simulink library "PC_Simulator_Lib"  (Simulink 8.2)
settings: Solver=ode45  StartTime=0.0  StopTime=10.0  RelTol=1e-3
values from neighbouring files (symbols this model uses):
  data = [r1 r2 r3 r4 L1 L2 L3 L4]    [strasse_Bedatung_HNI_ITI.m]
  distSameLane = 60    [InitialisationsEnv.m]
  eng_speed = [0 60 120 180 240 300 360 420 480 540 600 660 ... (101 elements, 1x101)]    [engine_table.mat]    (also in motor_parameter_calc.m = omega)
  Heading_init = 0    [Start.m]
  inertiaLateral = 25*(radiusWheel)^2    (= 4.129024)    [Start.m]
  laneWidth = 3.6    [InitialisationsEnv.m]    (also in strasse_Bedatung_HNI_ITI.m)
  omega_engine = [0.000000 150.000000 500.000000 1000.000000 1500.000000 2000.000000 2500.000000 3000.000000 3500.000000 4000.000000 4500.000000 5000.000000 5500.000000 6000.000000]    [friction_tables.m]
  omega_max = 6000    [engine_table.mat]    (also in motor_parameter_calc.m)
  omega_wheel = [0 20 40 60 80 100 122 143.7 164]    [friction_tables.m]
  para_Fellow_8_Points = ADAS.Fellow_8_Points    [ADAS_parameters.m]
  position_start_x = [x1 x2 x3 x4 x5 x6 x7]    [strasse_Bedatung_HNI_ITI.m]
  position_start_y = [y1 y2 y3 y4 y5 y6 y7]    [strasse_Bedatung_HNI_ITI.m]
  rad3rdLine = 57.2    [InitialisationsEnv.m]    (also in strasse_Bedatung_HNI_ITI.m)
  radiusWheel = 16*2.54/100    (= 0.4064)    [Start.m]
  s_values = [S1 S2 S3 S4 S5 S6 S7]    [strasse_Bedatung_HNI_ITI.m]
  segmentLimits = [segment1EndThirdLine                   segment2EndThirdLine                   segment3EndThirdLine                   segment4EndThirdLine                   segment5EndThirdLine                   segment6EndThirdLine                   segment7EndThirdLine                   segment8EndThirdLine                   ]    [InitialisationsEnv.m]    (also in strasse_Bedatung_HNI_ITI.m)
  setPosT = [-1.8 -5.4 -1.8 -5.4 -1.8 -5.4 -1.8 -5.4 -1.8 -5.4]    [InitialisationsEnv.m]
  torque = [297.089227105 300.997600937 304.800343044 308.497453426 312.088932082 315.574779014 318.95499422 322.229577701 325.398529457 328.461849487 331.419537793 334.271594373 ... (101 elements, 1x101)]    [engine_table.mat]    (also in motor_parameter_calc.m = g)
  Torque_lost = [0.000000 -8.777780 -15.000000 -26.800000 -29.600000 -32.700000 -35.900000 -39.300000 -42.800000 -46.500000 -50.300000 -54.300000 -58.500000 -62.800000 ]*0.6    [friction_tables.m]
  Torque_lost_wheel = [0.8 0.8 0.75 0.7 0.4 0.3 0.2 0.07 0.07]*0.2    [friction_tables.m]
  X_init = 0    [Start.m]
  Y_init = 1.8    [Start.m]
  Z_init = 0    [Start.m]
undefined symbols (not defined in the file or in its folder): Acc_Pedal, ADAS, Brake_Pedal, Joystick, Newton, Para, Raphson, Standard_Devices, Steering_Wheel_Angle, UDP_Protocol
libraries: simulink x43, rtwinlib x7, dspnetwork x2, simulink_extras x1, vrlib x1
(part 7 of 13)

== system PC_Simulator_Lib/Comunication_with_visualisation_normal_mode_new_Version/Subsystem2/Subsystem7 ==
  In1 : Inport
  Constant9 : Constant  Value=Z_init
  Sum : Sum  Inputs=|++
  Out1 : Outport
  wires:
  Sum/1 -> Out1/1
  Constant9/1 -> Sum/2
  In1/1 -> Sum/1

== system PC_Simulator_Lib/Comunication_with_visualisation_normal_mode_new_Version/Subsystem2/Subsystem8 ==
  In1 : Inport
  Constant9 : Constant  Value=Z_init
  Sum : Sum  Inputs=|++
  Out1 : Outport
  wires:
  In1/1 -> Sum/1
  Constant9/1 -> Sum/2
  Sum/1 -> Out1/1

== system PC_Simulator_Lib/Comunication_with_visualisation_normal_mode_new_Version/Subsystem2/Subsystem9 ==
  In1 : Inport
  Constant9 : Constant  Value=Z_init
  Sum : Sum  Inputs=|++
  Out1 : Outport
  wires:
  Sum/1 -> Out1/1
  Constant9/1 -> Sum/2
  In1/1 -> Sum/1

== system PC_Simulator_Lib/Drive_Train/4_Wheels_drive_train_and_Brake/Brake ==
  Feedback : Inport
  Add : Sum
  Bus Selector1 : BusSelector  OutputSignals=Vehicle_Dynamics.Vx_COG[m|s]
  Bus Selector6 : BusSelector  OutputSignals=ADAS.Brake_Pedal[norm]
  Compare To Constant : simulink/Logic and Bit Operations/Compare To Constant  relop=>=  const=0.7  OutDataTypeStr=uint8
  Compare To Constant1 : simulink/Logic and Bit Operations/Compare To Constant  relop=<=  const=-1  OutDataTypeStr=uint8
  Compare To Constant2 : simulink/Logic and Bit Operations/Compare To Constant  relop=<  const=0  OutDataTypeStr=uint8
  Constant1 : Constant  Value=0.35
  Constant2 : Constant
  Data Type Conversion : DataTypeConversion
  Data Type Conversion1 : DataTypeConversion
  Ground : Ground
  Ground1 : Ground
  Logical Operator : Logic  Operator=OR  AllPortsSameDT=off  OutDataTypeStr=boolean
  Product : Product  Inputs=5  RndMeth=Zero
  Product1 : Product  RndMeth=Zero
  Saturation : Saturate  UpperLimit=1  LowerLimit=0
  Sign : Signum
  Subsystem : Subsystem
  Subsystem1 : Subsystem
  Switch : Switch  Criteria=u2 > Threshold
  Terminator : Terminator
  Torque_max : Constant  Value=Para.DT.Torque_max_Brake.v
  Torque_Brake_Nm : Outport
  wires:
  Ground1/1 -> Subsystem/2(Omega_rad/s)
  Ground/1 -> Subsystem/1(Torque_Brake_Nm)
  Subsystem/1(Torque_Brake_act_Nm) -> Terminator/1
  Logical Operator/1 -> Data Type Conversion/1
  Compare To Constant/1 -> Logical Operator/1
  Bus Selector6/1 -> Saturation/1  "<Brake_Pedal[norm]>"
  Sign/1 -> Product/2
  Bus Selector1/1 -> Compare To Constant/1, Compare To Constant1/1, Subsystem1/1(v_X_CoG[m|s]), Compare To Constant2/1, Sign/1  "<Vx_COG[m|s]>"
  Feedback/1 -> Bus Selector1/1, Bus Selector6/1
  Torque_max/1 -> Product1/1
  Saturation/1 -> Product1/2, Subsystem1/2(Brake_Pedal[norm])
  Compare To Constant2/1 -> Data Type Conversion1/1
  Data Type Conversion1/1 -> Switch/2
  Constant1/1 -> Switch/1
  Product1/1 -> Product/1
  Switch/1 -> Product/4
  Constant2/1 -> Product/5, Switch/3
  Data Type Conversion/1 -> Product/3
  Compare To Constant1/1 -> Logical Operator/2
  Product/1 -> Add/1
  Add/1 -> Torque_Brake_Nm/1
  Subsystem1/1(Out1) -> Add/2

== system PC_Simulator_Lib/Drive_Train/4_Wheels_drive_train_and_Brake/FL ==
  F_z : Inport
  Vx : Inport  Port=2
  Vy : Inport  Port=3
  Coeffecient_of_friction : Inport  Port=4
  Torque_Drive_Nm : Inport  Port=5
  Torque_Brake_Nm : Inport  Port=6
  Alpha_Kappa_Selector2 : Subsystem
  Fx_calculator : MATLAB Function  TreatAsAtomicUnit=on
  Fy_calculator : MATLAB Function  TreatAsAtomicUnit=on
  Radius_of_tire : Constant  Value=radiusWheel
  Wheel dynamics : Subsystem
  Fx : Outport
  Fy : Outport  Port=2
  Omega : Outport  Port=3
  omegaDot_radPs2 : Outport  Port=4
  wires:
  Wheel dynamics/1(omega_radPs) -> Omega/1, Alpha_Kappa_Selector2/3(omega)
  Vx/1 -> Fy_calculator/3(V_x), Alpha_Kappa_Selector2/1(Vx)
  Radius_of_tire/1 -> Alpha_Kappa_Selector2/4(Rdyn)
  Vy/1 -> Alpha_Kappa_Selector2/2(Vy)
  F_z/1 -> Fy_calculator/4(Fz), Fx_calculator/3(Fz)
  Fy_calculator/1(Fy) -> Fy/1
  Coeffecient_of_friction/1 -> Fy_calculator/5(mue), Fx_calculator/4(mue)
  Fx_calculator/1(Fx) -> Wheel dynamics/1(F_x), Fx/1, Alpha_Kappa_Selector2/5(Fx)  "F_long"
  Wheel dynamics/2(omegaDot_radPs2) -> omegaDot_radPs2/1
  Torque_Drive_Nm/1 -> Wheel dynamics/2(Torque_Drive_Nm)
  Torque_Brake_Nm/1 -> Wheel dynamics/3(Torque_Brake_Nm)
  Alpha_Kappa_Selector2/1(kappa) -> Fx_calculator/1(lambda), Fy_calculator/1(lambda)
  Alpha_Kappa_Selector2/2(alpha) -> Fy_calculator/2(alpha), Fx_calculator/2(alpha)

== system PC_Simulator_Lib/Drive_Train/4_Wheels_drive_train_and_Brake/FR ==
  F_z : Inport
  Vx : Inport  Port=2
  Vy : Inport  Port=3
  Coeffecient_of_friction : Inport  Port=4
  Torque_Drive_Nm : Inport  Port=5
  Torque_Brake_Nm : Inport  Port=6
  Alpha_Kappa_Selector2 : Subsystem
  Fx_calculator : MATLAB Function  TreatAsAtomicUnit=on
  Fy_calculator : MATLAB Function  TreatAsAtomicUnit=on
  Radius_of_tire : Constant  Value=radiusWheel
  Wheel dynamics : Subsystem
  Fx : Outport
  Fy : Outport  Port=2
  Omega : Outport  Port=3
  omegaDot_radPs2 : Outport  Port=4
  wires:
  Wheel dynamics/1(omega_radPs) -> Alpha_Kappa_Selector2/3(omega), Omega/1
  Vx/1 -> Alpha_Kappa_Selector2/1(Vx), Fy_calculator/3(V_x)
  Radius_of_tire/1 -> Alpha_Kappa_Selector2/4(Rdyn)
  Vy/1 -> Alpha_Kappa_Selector2/2(Vy)
  F_z/1 -> Fy_calculator/4(Fz), Fx_calculator/3(Fz)
  Alpha_Kappa_Selector2/2(alpha) -> Fx_calculator/2(alpha), Fy_calculator/2(alpha)
  Alpha_Kappa_Selector2/1(kappa) -> Fy_calculator/1(lambda), Fx_calculator/1(lambda)
  Fy_calculator/1(Fy) -> Fy/1
  Coeffecient_of_friction/1 -> Fy_calculator/5(mue), Fx_calculator/4(mue)
  Fx_calculator/1(Fx) -> Alpha_Kappa_Selector2/5(Fx), Wheel dynamics/1(F_x), Fx/1  "F_long"
  Wheel dynamics/2(omegaDot_radPs2) -> omegaDot_radPs2/1
  Torque_Drive_Nm/1 -> Wheel dynamics/2(Torque_Drive_Nm)
  Torque_Brake_Nm/1 -> Wheel dynamics/3(Torque_Brake_Nm)

== system PC_Simulator_Lib/Drive_Train/4_Wheels_drive_train_and_Brake/RL ==
  F_z : Inport
  Vx : Inport  Port=2
  Vy : Inport  Port=3
  Coeffecient_of_friction : Inport  Port=4
  Torque_Drive_Nm : Inport  Port=5
  Torque_Brake_Nm : Inport  Port=6
  Alpha_Kappa_Selector2 : Subsystem
  Fx_calculator : MATLAB Function  TreatAsAtomicUnit=on
  Fy_calculator : MATLAB Function  TreatAsAtomicUnit=on
  Radius_of_tire : Constant  Value=radiusWheel
  Wheel dynamics : Subsystem
  Fx : Outport
  Fy : Outport  Port=2
  Omega : Outport  Port=3
  omegaDot_radPs2 : Outport  Port=4
  wires:
  Wheel dynamics/1(omega_radPs) -> Omega/1, Alpha_Kappa_Selector2/3(omega)
  Vx/1 -> Alpha_Kappa_Selector2/1(Vx), Fy_calculator/3(V_x)
  Radius_of_tire/1 -> Alpha_Kappa_Selector2/4(Rdyn)
  Vy/1 -> Alpha_Kappa_Selector2/2(Vy)
  F_z/1 -> Fy_calculator/4(Fz), Fx_calculator/3(Fz)
  Alpha_Kappa_Selector2/2(alpha) -> Fx_calculator/2(alpha), Fy_calculator/2(alpha)
  Alpha_Kappa_Selector2/1(kappa) -> Fy_calculator/1(lambda), Fx_calculator/1(lambda)
  Fy_calculator/1(Fy) -> Fy/1
  Coeffecient_of_friction/1 -> Fy_calculator/5(mue), Fx_calculator/4(mue)
  Fx_calculator/1(Fx) -> Wheel dynamics/1(F_x), Fx/1, Alpha_Kappa_Selector2/5(Fx)  "F_long"
  Wheel dynamics/2(omegaDot_radPs2) -> omegaDot_radPs2/1
  Torque_Drive_Nm/1 -> Wheel dynamics/2(Torque_Drive_Nm)
  Torque_Brake_Nm/1 -> Wheel dynamics/3(Torque_Brake_Nm)

== system PC_Simulator_Lib/Drive_Train/4_Wheels_drive_train_and_Brake/RR ==
  F_z : Inport
  Vx : Inport  Port=2
  Vy : Inport  Port=3
  Coeffecient_of_friction : Inport  Port=4
  Torque_Drive_Nm : Inport  Port=5
  Torque_Brake_Nm : Inport  Port=6
  Alpha_Kappa_Selector2 : Subsystem
  Fx_calculator : MATLAB Function  TreatAsAtomicUnit=on
  Fy_calculator : MATLAB Function  TreatAsAtomicUnit=on
  Radius_of_tire : Constant  Value=radiusWheel
  Wheel dynamics : Subsystem
  Fx : Outport
  Fy : Outport  Port=2
  Omega : Outport  Port=3
  omegaDot_radPs2 : Outport  Port=4
  wires:
  Wheel dynamics/1(omega_radPs) -> Omega/1, Alpha_Kappa_Selector2/3(omega)
  Vx/1 -> Fy_calculator/3(V_x), Alpha_Kappa_Selector2/1(Vx)
  Radius_of_tire/1 -> Alpha_Kappa_Selector2/4(Rdyn)
  Vy/1 -> Alpha_Kappa_Selector2/2(Vy)
  F_z/1 -> Fy_calculator/4(Fz), Fx_calculator/3(Fz)
  Alpha_Kappa_Selector2/2(alpha) -> Fx_calculator/2(alpha), Fy_calculator/2(alpha)
  Alpha_Kappa_Selector2/1(kappa) -> Fy_calculator/1(lambda), Fx_calculator/1(lambda)
  Fy_calculator/1(Fy) -> Fy/1
  Coeffecient_of_friction/1 -> Fy_calculator/5(mue), Fx_calculator/4(mue)
  Fx_calculator/1(Fx) -> Wheel dynamics/1(F_x), Fx/1, Alpha_Kappa_Selector2/5(Fx)  "F_long"
  Wheel dynamics/2(omegaDot_radPs2) -> omegaDot_radPs2/1
  Torque_Drive_Nm/1 -> Wheel dynamics/2(Torque_Drive_Nm)
  Torque_Brake_Nm/1 -> Wheel dynamics/3(Torque_Brake_Nm)

== system PC_Simulator_Lib/Environment/Environment_Model/Master driver ==
  setVelS[km/h] : Inport
  setPosT[m] : Inport  Port=2
  actualPosS[m] : Inport  Port=3
  actualPosT[m] : Inport  Port=4
  actualVelS[m/s] : Inport  Port=5
  distSameLanes[m] : Inport  Port=6
  mainCarPosS[m] : Inport  Port=7
  mainCarPosT[m] : Inport  Port=8
  mainCarVelS[m/s] : Inport  Port=9
  mainCarWidth[m] : Inport  Port=10
  masterDriver : MATLAB Function  TreatAsAtomicUnit=on
  desiredVelS[km/h] : Outport
  desiredPosT[m] : Outport  Port=2
  wires:
  masterDriver/2(desiredPosT) -> desiredPosT[m]/1
  masterDriver/1(desiredVelS) -> desiredVelS[km/h]/1
  mainCarPosS[m]/1 -> masterDriver/7(mainCarPosS)
  distSameLanes[m]/1 -> masterDriver/6(distSameLanes)
  actualVelS[m/s]/1 -> masterDriver/5(actualVelS)
  actualPosT[m]/1 -> masterDriver/4(actualPosT)
  actualPosS[m]/1 -> masterDriver/3(actualPosS)
  setPosT[m]/1 -> masterDriver/2(setPosT)
  setVelS[km/h]/1 -> masterDriver/1(setVelS)
  mainCarPosT[m]/1 -> masterDriver/8(mainCarPosT)
  mainCarVelS[m/s]/1 -> masterDriver/9(mainCarVelS)
  mainCarWidth[m]/1 -> masterDriver/10(mainCarWidth)

== system PC_Simulator_Lib/Environment/Environment_Model/Road model ==
  note: Simple road model to transform the (s,t) point of the
      | local coordinate system to (x,y) point of the global
      | coordinate system
  note: Road model to transform
      | the (s,t) point to (x,y) point
  s[m] : Inport
  t[m] : Inport  Port=2
  segmentLimits[m] : Inport  Port=3
  laneWidth[m] : Inport  Port=4
  rad3rdLine[m] : Inport  Port=5
  st_xy : MATLAB Function  TreatAsAtomicUnit=on
  x[m] : Outport
  y[m] : Outport  Port=2
  z[m] : Outport  Port=3
  headingAngle[deg] : Outport  Port=4
  wires:
  st_xy/4(headingAngle) -> headingAngle[deg]/1
  st_xy/3(z) -> z[m]/1
  st_xy/2(y) -> y[m]/1
  st_xy/1(x) -> x[m]/1
  rad3rdLine[m]/1 -> st_xy/5(rad3rdLine)
  laneWidth[m]/1 -> st_xy/4(laneWidth)
  segmentLimits[m]/1 -> st_xy/3(segmentLimits)
  t[m]/1 -> st_xy/2(t)
  s[m]/1 -> st_xy/1(s)

== system PC_Simulator_Lib/Environment/Environment_Model/Subsystem ==
  v_relative_Sensor[m|s] : Inport
  1-D Lookup Table1 : Lookup_n-D  NumberOfTableDimensions=1  BreakpointsForDimension1=ADAS.EBA.Braking_Distance_LookUpTable.velocity  BeginIndexSearchUsingPreviousIndexResult=on  Table=ADAS.EBA.Braking_Distance_LookUpTable.Distance  InternalRulePriority=Speed  RndMeth=Simplest  InputSameDT=on
  Abs : Abs
  Divide : Product  Inputs=/*
  Gain : Gain  Gain=3.6
  Math Function : Math  Operator=square  SaturateOnIntegerOverflow=on
  Braking_Distance[m] : Outport
  wires:
  v_relative_Sensor[m|s]/1 -> Abs/1, Math Function/1
  Math Function/1 -> Divide/2
  Divide/1 -> Braking_Distance[m]/1
  Gain/1 -> 1-D Lookup Table1/1
  1-D Lookup Table1/1 -> Divide/1
  Abs/1 -> Gain/1

== system PC_Simulator_Lib/Environment/Environment_Model/Traffic_Vehicle_Model1 ==
  ResetSig[] : Inport
  VelSDesired : Inport  Port=2
  Vehicle_Model_s : Subsystem
  VelS[m/s] : Outport
  PosS[m] : Outport  Port=2
  wires:
  Vehicle_Model_s/1(VelS[m/s]) -> VelS[m/s]/1
  Vehicle_Model_s/2(PosS[m]) -> PosS[m]/1
  ResetSig[]/1 -> Vehicle_Model_s/1(ResetSig[])
  VelSDesired/1 -> Vehicle_Model_s/2(VelSDesired[Km/h])

== system PC_Simulator_Lib/Environment/Environment_Model/Traffic_Vehicle_Model11 ==
  ResetSig[] : Inport
  VelSDesired[km/h] : Inport  Port=2
  PosTDesired[m] : Inport  Port=3
  Vehicle_Model_s : Subsystem
  Vehicle_Model_t : Subsystem
  VelS[m/s] : Outport
  PosS[m] : Outport  Port=2
  PosT[m] : Outport  Port=3
  wires:
  PosTDesired[m]/1 -> Vehicle_Model_t/2(PosTDesired[m])
  Vehicle_Model_t/1(PosT[m]) -> PosT[m]/1
  VelSDesired[km/h]/1 -> Vehicle_Model_s/2(VelSDesired[Km/h])
  ResetSig[]/1 -> Vehicle_Model_t/1(ResetSig[]), Vehicle_Model_s/1(ResetSig[])
  Vehicle_Model_s/2(PosS[m]) -> PosS[m]/1
  Vehicle_Model_s/1(VelS[m/s]) -> VelS[m/s]/1

== system PC_Simulator_Lib/Environment/Environment_Model/Traffic_Vehicle_Model2 ==
  ResetSig[] : Inport
  VelSDesired : Inport  Port=2
  Vehicle_Model_s : Subsystem
  VelS[m/s] : Outport
  PosS[m] : Outport  Port=2
  wires:
  Vehicle_Model_s/1(VelS[m/s]) -> VelS[m/s]/1
  Vehicle_Model_s/2(PosS[m]) -> PosS[m]/1
  ResetSig[]/1 -> Vehicle_Model_s/1(ResetSig[])
  VelSDesired/1 -> Vehicle_Model_s/2(VelSDesired[Km/h])

== system PC_Simulator_Lib/Environment/Environment_Model/Traffic_Vehicle_Model3 ==
  ResetSig[] : Inport
  VelSDesired : Inport  Port=2
  Vehicle_Model_s : Subsystem
  VelS[m/s] : Outport
  PosS[m] : Outport  Port=2
  wires:
  Vehicle_Model_s/1(VelS[m/s]) -> VelS[m/s]/1
  Vehicle_Model_s/2(PosS[m]) -> PosS[m]/1
  ResetSig[]/1 -> Vehicle_Model_s/1(ResetSig[])
  VelSDesired/1 -> Vehicle_Model_s/2(VelSDesired[Km/h])

== system PC_Simulator_Lib/Environment/Environment_Model/Traffic_Vehicle_Model4 ==
  ResetSig[] : Inport
  VelSDesired : Inport  Port=2
  Vehicle_Model_s : Subsystem
  VelS[m/s] : Outport
  PosS[m] : Outport  Port=2
  wires:
  Vehicle_Model_s/1(VelS[m/s]) -> VelS[m/s]/1
  Vehicle_Model_s/2(PosS[m]) -> PosS[m]/1
  ResetSig[]/1 -> Vehicle_Model_s/1(ResetSig[])
  VelSDesired/1 -> Vehicle_Model_s/2(VelSDesired[Km/h])

== system PC_Simulator_Lib/Environment/Environment_Model/Traffic_Vehicle_Model5 ==
  ResetSig[] : Inport
  VelSDesired : Inport  Port=2
  Vehicle_Model_s : Subsystem
  VelS[m/s] : Outport
  PosS[m] : Outport  Port=2
  wires:
  Vehicle_Model_s/1(VelS[m/s]) -> VelS[m/s]/1
  Vehicle_Model_s/2(PosS[m]) -> PosS[m]/1
  ResetSig[]/1 -> Vehicle_Model_s/1(ResetSig[])
  VelSDesired/1 -> Vehicle_Model_s/2(VelSDesired[Km/h])

== system PC_Simulator_Lib/Environment/Environment_Model/Traffic_Vehicle_Model6 ==
  ResetSig[] : Inport
  VelSDesired : Inport  Port=2
  Vehicle_Model_s : Subsystem
  VelS[m/s] : Outport
  PosS[m] : Outport  Port=2
  wires:
  Vehicle_Model_s/1(VelS[m/s]) -> VelS[m/s]/1
  Vehicle_Model_s/2(PosS[m]) -> PosS[m]/1
  ResetSig[]/1 -> Vehicle_Model_s/1(ResetSig[])
  VelSDesired/1 -> Vehicle_Model_s/2(VelSDesired[Km/h])

== system PC_Simulator_Lib/Environment/Environment_Model/Traffic_Vehicle_Model7 ==
  ResetSig[] : Inport
  VelSDesired : Inport  Port=2
  Vehicle_Model_s : Subsystem
  VelS[m/s] : Outport
  PosS[m] : Outport  Port=2
  wires:
  Vehicle_Model_s/1(VelS[m/s]) -> VelS[m/s]/1
  Vehicle_Model_s/2(PosS[m]) -> PosS[m]/1
  ResetSig[]/1 -> Vehicle_Model_s/1(ResetSig[])
  VelSDesired/1 -> Vehicle_Model_s/2(VelSDesired[Km/h])

== system PC_Simulator_Lib/Environment/Environment_Model/Traffic_Vehicle_Model8 ==
  ResetSig[] : Inport
  VelSDesired : Inport  Port=2
  Vehicle_Model_s : Subsystem
  VelS[m/s] : Outport
  PosS[m] : Outport  Port=2
  wires:
  Vehicle_Model_s/1(VelS[m/s]) -> VelS[m/s]/1
  Vehicle_Model_s/2(PosS[m]) -> PosS[m]/1
  ResetSig[]/1 -> Vehicle_Model_s/1(ResetSig[])
  VelSDesired/1 -> Vehicle_Model_s/2(VelSDesired[Km/h])

== system PC_Simulator_Lib/Environment/Environment_Model/Traffic_Vehicle_Model9 ==
  ResetSig[] : Inport
  VelSDesired : Inport  Port=2
  Vehicle_Model_s : Subsystem
  VelS[m/s] : Outport
  PosS[m] : Outport  Port=2
  wires:
  Vehicle_Model_s/1(VelS[m/s]) -> VelS[m/s]/1
  Vehicle_Model_s/2(PosS[m]) -> PosS[m]/1
  ResetSig[]/1 -> Vehicle_Model_s/1(ResetSig[])
  VelSDesired/1 -> Vehicle_Model_s/2(VelSDesired[Km/h])

== system PC_Simulator_Lib/Environment/Maping_Input /Strasse_xy ==
  x[m] : Inport
  y[m] : Inport  Port=2
  Constant : Constant  Value=data
  Constant1 : Constant  Value=position_start_x
  Constant2 : Constant  Value=position_start_y
  Constant3 : Constant  Value=s_values
  Embedded MATLAB Function : MATLAB Function  TreatAsAtomicUnit=on
  Terminator2 : Terminator
  Terminator3 : Terminator
  s[m] : Outport
  t[m] : Outport  Port=2
  Heading_angle[rad] : Outport  Port=3
  wires:
  Constant/1 -> Embedded MATLAB Function/1(data)
  Constant1/1 -> Embedded MATLAB Function/2(position_start_x)
  Constant2/1 -> Embedded MATLAB Function/3(position_start_y)
  Constant3/1 -> Embedded MATLAB Function/4(s_values)
  Embedded MATLAB Function/3(mue) -> Terminator2/1
  Embedded MATLAB Function/1(z) -> Terminator3/1
  x[m]/1 -> Embedded MATLAB Function/5(x)
  y[m]/1 -> Embedded MATLAB Function/6(y)
  Embedded MATLAB Function/4(s) -> s[m]/1
  Embedded MATLAB Function/5(t) -> t[m]/1
  Embedded MATLAB Function/2(psi) -> Heading_angle[rad]/1

== system PC_Simulator_Lib/Environment/Maping_Output /Subsystem ==
  x_fellows_Vector[m] : Inport
  y_fellows_Vector[m] : Inport  Port=2
  z_fellows_Vector[m] : Inport  Port=3
  Heading_fellows_Vector[deg] : Inport  Port=4
  S_Velocity_Vector[m|s] : Inport  Port=5
  Bus Creator{1..4,6} (5 alike) : BusCreator  Inputs=10
  Bus Creator5 : BusCreator  Inputs=5
  Constant : Constant  Value=0
  Demux{,1..4} (5 alike) : Demux  Outputs=10
  Terminator : Terminator
  Fellows_Pos_Oriantation_Bus : Outport
  wires:
  [yaw_smart_car] -> Bus Creator4/10  "Heading_fellow10[deg]"
  Bus Creator3/1 -> Bus Creator5/1  "x_fellows_vector"
  x_fellows_Vector[m]/1 -> Demux/1
  Demux/1 -> Bus Creator3/1  "x_fellow1[m]"
  Demux/2 -> Bus Creator3/2  "x_fellow2[m]"
  Demux/3 -> Bus Creator3/3  "x_fellow3[m]"
  Demux/4 -> Bus Creator3/4  "x_fellow4[m]"
  Demux/5 -> Bus Creator3/5  "x_fellow5[m]"
  Demux/6 -> Bus Creator3/6  "x_fellow6[m]"
  Demux/7 -> Bus Creator3/7  "x_fellow7[m]"
  Demux/8 -> Bus Creator3/8  "x_fellow8[m]"
  Demux/9 -> Bus Creator3/9  "x_fellow9[m]"
  Demux/10 -> Bus Creator3/10  "x_fellow10[m]"
  Bus Creator1/1 -> Bus Creator5/2  "y_fellows_vector"
  y_fellows_Vector[m]/1 -> Demux1/1
  Demux1/1 -> Bus Creator1/1  "y_fellow1[m]"
  Demux1/2 -> Bus Creator1/2  "y_fellow2[m]"
  Demux1/3 -> Bus Creator1/3  "y_fellow3[m]"
  Demux1/4 -> Bus Creator1/4  "y_fellow4[m]"
  Demux1/5 -> Bus Creator1/5  "y_fellow5[m]"
  Demux1/6 -> Bus Creator1/6  "y_fellow6[m]"
  Demux1/7 -> Bus Creator1/7  "y_fellow7[m]"
  Demux1/8 -> Bus Creator1/8  "y_fellow8[m]"
  Demux1/9 -> Bus Creator1/9  "y_fellow9[m]"
  Demux1/10 -> Bus Creator1/10  "y_fellow10[m]"
  Bus Creator2/1 -> Bus Creator5/3  "z_fellows_vector"
  z_fellows_Vector[m]/1 -> Demux2/1
  Demux2/1 -> Bus Creator2/1  "z_fellow1[m]"
  Demux2/2 -> Bus Creator2/2  "z_fellow2[m]"
  Demux2/3 -> Bus Creator2/3  "z_fellow3[m]"
  Demux2/4 -> Bus Creator2/4  "z_fellow4[m]"
  Demux2/5 -> Bus Creator2/5  "z_fellow5[m]"
  Demux2/6 -> Bus Creator2/6  "z_fellow6[m]"
  Demux2/7 -> Bus Creator2/7  "z_fellow7[m]"
  Demux2/8 -> Bus Creator2/8  "z_fellow8[m]"
  Demux2/9 -> Bus Creator2/9  "z_fellow9[m]"
  Demux2/10 -> Bus Creator2/10  "z_fellow10[m]"
  Bus Creator4/1 -> Bus Creator5/4  "Heading_fellows_vector"
  Heading_fellows_Vector[deg]/1 -> Demux3/1
  Demux3/1 -> Bus Creator4/1  "Heading_fellow1[deg]"
  Demux3/2 -> Bus Creator4/2  "Heading_fellow2[deg]"
  Demux3/3 -> Bus Creator4/3  "Heading_fellow3[deg]"
  Demux3/4 -> Bus Creator4/4  "Heading_fellow4[deg]"
  Demux3/5 -> Bus Creator4/5  "Heading_fellow5[deg]"
  Demux3/6 -> Bus Creator4/6  "Heading_fellow6[deg]"
  Demux3/7 -> Bus Creator4/7  "Heading_fellow7[deg]"
  Demux3/8 -> Bus Creator4/8  "Heading_fellow8[deg]"
  Demux3/9 -> Bus Creator4/9  "Heading_fellow9[deg]"
  Demux3/10 -> Terminator/1  "Heading_fellow10[deg]"
  Bus Creator5/1 -> Fellows_Pos_Oriantation_Bus/1
  Bus Creator6/1 -> Bus Creator5/5  "velocity_fellows_vector[m|s]"
  S_Velocity_Vector[m|s]/1 -> Demux4/1
  Demux4/1 -> Bus Creator6/1  "velocity_fellow1[m|s]"
  Demux4/2 -> Bus Creator6/2  "velocity_fellow2[m|s]"
  Demux4/3 -> Bus Creator6/3  "velocity_fellow3[m|s]"
  Demux4/4 -> Bus Creator6/4  "velocity_fellow4[m|s]"
  Demux4/5 -> Bus Creator6/5  "velocity_fellow5[m|s]"
  Demux4/6 -> Bus Creator6/6  "velocity_fellow6[m|s]"
  Demux4/7 -> Bus Creator6/7  "velocity_fellow7[m|s]"
  Demux4/8 -> Bus Creator6/8  "velocity_fellow8[m|s]"
  Demux4/9 -> Bus Creator6/9  "velocity_fellow9[m|s]"
  Demux4/10 -> Bus Creator6/10  "velocity_fellow10[m|s]"

== system PC_Simulator_Lib/HMI_Realtime/HMI_Logitech1/Subsystem1 ==
  In1 : Inport
  Compare To Constant : simulink/Logic and Bit Operations/Compare To Constant  relop=>=  const=0.0001  OutDataTypeStr=boolean
  Constant : Constant
  Data Type Conversion : DataTypeConversion
  Gain : Gain  Gain=0.5
  Product : Product
  Sum : Sum  Inputs=|-+
  Out1 : Outport
  wires:
  Gain/1 -> Compare To Constant/1, Product/1
  Constant/1 -> Sum/2
  Sum/1 -> Gain/1
  In1/1 -> Sum/1
  Product/1 -> Out1/1
  Compare To Constant/1 -> Data Type Conversion/1
  Data Type Conversion/1 -> Product/2

== system PC_Simulator_Lib/HMI_Realtime/HMI_Logitech1/Subsystem2 ==
  In1 : Inport
  Compare To Constant : simulink/Logic and Bit Operations/Compare To Constant  relop=>=  const=0.0001  OutDataTypeStr=boolean
  Constant : Constant
  Data Type Conversion : DataTypeConversion
  Gain : Gain  Gain=0.5
  Product : Product
  Sum : Sum  Inputs=|-+
  Out1 : Outport
  wires:
  Gain/1 -> Compare To Constant/1, Product/1
  Constant/1 -> Sum/2
  Sum/1 -> Gain/1
  In1/1 -> Sum/1
  Product/1 -> Out1/1
  Compare To Constant/1 -> Data Type Conversion/1
  Data Type Conversion/1 -> Product/2

== system PC_Simulator_Lib/HMI_Realtime_normal_mode/HMI_Logitech/Subsystem2 ==
  In1 : Inport
  Constant : Constant
  Gain : Gain  Gain=0.5
  Sum : Sum  Inputs=|-+
  Out1 : Outport
  wires:
  Gain/1 -> Out1/1
  Constant/1 -> Sum/2
  Sum/1 -> Gain/1
  In1/1 -> Sum/1

== system PC_Simulator_Lib/HMI_Realtime_normal_mode/HMI_Logitech/Subsystem3 ==
  In1 : Inport
  Constant : Constant
  Gain : Gain  Gain=0.5
  Sum : Sum  Inputs=|-+
  Out1 : Outport
  wires:
  Gain/1 -> Out1/1
  In1/1 -> Sum/1
  Sum/1 -> Gain/1
  Constant/1 -> Sum/2

== system PC_Simulator_Lib/Vehicle dynamics/Forces_transformation/Force_of_Aerodynamics ==
  note: Neglecting the air resistance effect in Y and modefing the equation
      | (V_abs*cos(slip))^2*Cd
      | insted of
      | V_abs^2*cos(slip)*Cd
      | by Berry
      | if not understud call me now
      | +20122299183
  velocity_of_car_absolut : Inport
  Slip_angle_of_velocity : Inport  Port=2
  Demux : Demux  Outputs=2
  Gain : Gain  Gain=Para.VD.Air_Risistance_Coefficient.v
  Product1 : Product  RndMeth=Zero
  Product2 : Product  RndMeth=Zero
  Product4 : Product  RndMeth=Zero
  Trigonometric Function3 : Trigonometry  Operator=cos
  Unary Minus : UnaryMinus
  Force_of_aerodynamics_in_X : Outport
  wires:
  Trigonometric Function3/1 -> Product4/2
  Slip_angle_of_velocity/1 -> Trigonometric Function3/1
  Product4/1 -> Product1/2, Product1/1
  Product1/1 -> Gain/1
  velocity_of_car_absolut/1 -> Demux/1
  Demux/1 -> Product4/1
  Demux/2 -> Unary Minus/1
  Unary Minus/1 -> Product2/2
  Gain/1 -> Product2/1
  Product2/1 -> Force_of_aerodynamics_in_X/1

== system PC_Simulator_Lib/Vehicle dynamics/Forces_transformation/Moment _about _Z_axis_calculation ==
  note: FL_X
  note: FR_X
  note: RL_X
  note: RR_X
  note: FL_Y
  note: FR_Y
  note: RL_Y
  note: RR_Y
  note: produce
      | the moment around Z
      | axis due to the total effect
      | of the forces acting on the
      | vehicle
  Forces_Acting_in_X_Wheels : Inport
  Forces_Acting_in_Y_Wheels : Inport  Port=2
  Add : Sum  Inputs=-++-
  Demux1 : Demux
  Demux3 : Demux
  Length_CG_Front_Wheels : Constant  Value=Para.VD.Length_Front.v
  Length_CG_Rear_Wheels : Constant  Value=Para.VD.Length_Rear.v
  Product{1..4} (4 alike) : Product  RndMeth=Zero
  Subtract{1..4} (4 alike) : Sum
  Width_of_Car/2 : Constant  Value=Para.VD.Wheel_Base_Width.v/2
  Moment _about _Z_axis : Outport
  wires:
  Demux1/1 -> Subtract2/1
  Demux1/2 -> Subtract2/2
  Subtract2/1 -> Product1/1
  Demux1/3 -> Subtract1/1
  Demux1/4 -> Subtract1/2
  Subtract1/1 -> Product2/1
  Product1/1 -> Add/3
  Product2/1 -> Add/4
  Product3/1 -> Add/1
  Product4/1 -> Add/2
  Subtract3/1 -> Product4/2
  Subtract4/1 -> Product3/2
  Demux3/1 -> Subtract4/1
  Demux3/4 -> Subtract3/2
  Width_of_Car/2/1 -> Product3/1, Product4/1
  Forces_Acting_in_X_Wheels/1 -> Demux3/1
  Forces_Acting_in_Y_Wheels/1 -> Demux1/1
  Length_CG_Front_Wheels/1 -> Product1/2
  Length_CG_Rear_Wheels/1 -> Product2/2
  Demux3/3 -> Subtract4/2
  Demux3/2 -> Subtract3/1
  Add/1 -> Moment _about _Z_axis/1

== system PC_Simulator_Lib/Vehicle dynamics/Forces_transformation/Moment _about _x_axis_calculation ==
  note: FL_Z
  note: FR_Z
  note: RL_Z
  note: RR_Z
  note: FL_Y
  note: FR_Y
  note: RL_Y
  note: RR_Y
  note: the total effect of forces
      | acting as a moment
      | around the X axis
  Forces_Z_Wheels : Inport
  Forces_Y_Wheels : Inport  Port=2
  Hight_Front_Left : Inport  Port=3
  Hight_Front_Right : Inport  Port=4
  Hight_Rear_Left : Inport  Port=5
  Hight_Rear_Right : Inport  Port=6
  Add1 : Sum  Inputs=+-+-
  Add2 : Sum  Inputs=++++
  Add3 : Sum
  Demux2 : Demux
  Demux3 : Demux
  Divide{9..16} (8 alike) : Product  Inputs=**
  Width_of_Car/1 : Constant  Value=Para.VD.Wheel_Base_Width.v/2
  Moment _about _X_axis1 : Outport
  wires:
  Divide12/1 -> Add1/4
  Divide11/1 -> Add1/3
  Divide10/1 -> Add1/2
  Divide9/1 -> Add1/1
  Width_of_Car/1/1 -> Divide9/1, Divide10/1, Divide11/1, Divide12/1
  Demux2/1 -> Divide9/2
  Demux2/2 -> Divide10/2
  Demux2/3 -> Divide11/2
  Demux2/4 -> Divide12/2
  Forces_Z_Wheels/1 -> Demux2/1
  Divide13/1 -> Add2/1
  Divide14/1 -> Add2/2
  Divide15/1 -> Add2/3
  Divide16/1 -> Add2/4
  Demux3/1 -> Divide13/1
  Demux3/2 -> Divide14/1
  Demux3/3 -> Divide15/1
  Demux3/4 -> Divide16/1
  Forces_Y_Wheels/1 -> Demux3/1
  Hight_Front_Left/1 -> Divide13/2
  Hight_Front_Right/1 -> Divide14/2
  Hight_Rear_Left/1 -> Divide15/2
  Hight_Rear_Right/1 -> Divide16/2
  Add1/1 -> Add3/1
  Add2/1 -> Add3/2
  Add3/1 -> Moment _about _X_axis1/1

== system PC_Simulator_Lib/Vehicle dynamics/Forces_transformation/Moment _about _y_axis_calculation ==
  note: FL_Z
  note: FR_Z
  note: RL_Z
  note: RR_Z
  note: FL_X
  note: FR_X
  note: RL_X
  note: RR_X
  note: the total effect of the car forces
      | represented as a moment acting on the
      | CG around Y axis
  Forces_Z_Wheels : Inport
  Forces_X_Wheels : Inport  Port=2
  Hight_Front_Left : Inport  Port=3
  Hight_Front_Right : Inport  Port=4
  Hight_Rear_Left : Inport  Port=5
  Hight_Rear_Right : Inport  Port=6
  Add1 : Sum  Inputs=--++
  Add2 : Sum  Inputs=----
  Add3 : Sum
  Demux1 : Demux
  Demux9 : Demux
  Divide{8..15} (8 alike) : Product  Inputs=**
  Length_CG_Front_Wheels : Constant  Value=Para.VD.Length_Front.v
  Length_CG_Rear_Wheels : Constant  Value=Para.VD.Length_Rear.v
  Moment _about _Y_axis2 : Outport
  wires:
  Add1/1 -> Add3/1
  Add2/1 -> Add3/2
  Divide8/1 -> Add1/1
  Divide9/1 -> Add1/2
  Divide10/1 -> Add1/3
  Divide11/1 -> Add1/4
  Divide12/1 -> Add2/1
  Divide13/1 -> Add2/2
  Divide14/1 -> Add2/3
  Divide15/1 -> Add2/4
  Demux9/1 -> Divide8/1
  Demux9/2 -> Divide9/1
  Demux9/3 -> Divide10/1
  Demux9/4 -> Divide11/1
  Length_CG_Front_Wheels/1 -> Divide8/2, Divide9/2
  Length_CG_Rear_Wheels/1 -> Divide10/2, Divide11/2
  Forces_Z_Wheels/1 -> Demux9/1
  Demux1/1 -> Divide12/1
  Demux1/2 -> Divide13/1
  Demux1/3 -> Divide14/1
  Demux1/4 -> Divide15/1
  Forces_X_Wheels/1 -> Demux1/1
  Hight_Front_Left/1 -> Divide12/2
  Hight_Front_Right/1 -> Divide13/2
  Hight_Rear_Left/1 -> Divide14/2
  Hight_Rear_Right/1 -> Divide15/2
  Add3/1 -> Moment _about _Y_axis2/1

== system PC_Simulator_Lib/Vehicle dynamics/Forces_transformation/Z1-->angles ==
  Z1(4) : Inport
  Constant3 : Constant  Value=-2*Para.VD.Length_Front.v
  Constant4 : Constant  Value=Para.VD.Wheel_Base_Width.v
  Demux : Demux
  Divide : Product  Inputs=*/
  Divide1 : Product  Inputs=*/
  Subtract3 : Sum  Inputs=+-
  Subtract4 : Sum  Inputs=+-
  Terminator : Terminator
  Trigonometric Function1 : Trigonometry  Operator=asin
  Trigonometric Function2 : Trigonometry  Operator=asin
  Roll_angel(z1)1 : Outport
  Pitch_angel(z1) : Outport  Port=2
  wires:
  Trigonometric Function2/1 -> Roll_angel(z1)1/1
  Divide1/1 -> Trigonometric Function2/1
  Constant4/1 -> Divide1/2
  Subtract4/1 -> Divide1/1
  Demux/2 -> Subtract4/2
  Trigonometric Function1/1 -> Pitch_angel(z1)/1
  Divide/1 -> Trigonometric Function1/1
  Constant3/1 -> Divide/2
  Subtract3/1 -> Divide/1
  Demux/3 -> Subtract3/2
  Demux/1 -> Subtract4/1, Subtract3/1
  Z1(4)/1 -> Demux/1
  Demux/4 -> Terminator/1

== system PC_Simulator_Lib/Vehicle dynamics/Forces_transformation/force acting in X direction ==
  note: Force_Front_Left_in_x
  note: Force_Front_Right_in_x
  note: Force_rear_left_in_x
  note: Force_rear_right_in_x
  note: the summation of forces
      | acting on the X direction
      | on CG
  Forces_Acting_In_X_Wheel : Inport
  Force_acting_in_x_from_mass : Inport  Port=2
  Force_in_x_air : Inport  Port=3
  Add : Sum  Inputs=++++++
  Demux1 : Demux
  Force_acting_on_CG_in_x : Outport
  wires:
  Demux1/1 -> Add/1
  Demux1/2 -> Add/2
  Demux1/3 -> Add/3
  Demux1/4 -> Add/4
  Force_acting_in_x_from_mass/1 -> Add/5
  Force_in_x_air/1 -> Add/6
  Forces_Acting_In_X_Wheel/1 -> Demux1/1
  Add/1 -> Force_acting_on_CG_in_x/1

== system PC_Simulator_Lib/Vehicle dynamics/Forces_transformation/force acting in Y direction ==
  note: Force_Front_Left_in_Y
  note: Force_Front_Right_in_Y
  note: Force_Rear_Left_in_Y
  note: Force_Rear_Right_in_Y
  note: the summation of forces
      | acting on the Y direction
      | on CG
  Forces_Acting_In_Y_Wheels : Inport
  Force_From_Mass_Y : Inport  Port=2
  Add : Sum  Inputs=+++++
  Demux2 : Demux
  Force_acting_on_CG_in_Y : Outport
  wires:
  Force_From_Mass_Y/1 -> Add/5
  Demux2/4 -> Add/4
  Demux2/3 -> Add/3
  Demux2/2 -> Add/2
  Demux2/1 -> Add/1
  Forces_Acting_In_Y_Wheels/1 -> Demux2/1
  Add/1 -> Force_acting_on_CG_in_Y/1

== system PC_Simulator_Lib/Vehicle dynamics/Forces_transformation/force acting in Z direction ==
  note: the summation of forces acting
      | on CG in Z direction
  Forces_Z_Wheel : Inport
  Force_Mass_Z : Inport  Port=2
  Add : Sum  Inputs=+++++
  Demux5 : Demux
  Force_acting_on_CG_in_z : Outport
  wires:
  Demux5/1 -> Add/1
  Demux5/2 -> Add/2
  Demux5/3 -> Add/3
  Add/1 -> Force_acting_on_CG_in_z/1
  Demux5/4 -> Add/4
  Force_Mass_Z/1 -> Add/5
  Forces_Z_Wheel/1 -> Demux5/1

== system PC_Simulator_Lib/Vehicle dynamics/Forces_transformation/inclination_effect_on_mass ==
  note: FZ_due to roll
  Roll_angle(z1) : Inport
  Pitch_angel(z1) : Inport  Port=2
  Gain : Gain  Gain=-1
  Gain1 : Gain  Gain=-1
  Product{1..4} (4 alike) : Product  RndMeth=Zero
  Trigonometric Function : Trigonometry  Operator=cos
  Trigonometric Function1 : Trigonometry  Operator=cos
  Trigonometric Function2 : Trigonometry
  Trigonometric Function3 : Trigonometry
  m * g : Constant  Value=Para.VD.Mass.v * Para.VD.gravity.v
  FZ_due_to_mass : Outport
  Fx_due_to_mass : Outport  Port=2
  Fy_due_to_mass : Outport  Port=3
  wires:
  Pitch_angel(z1)/1 -> Trigonometric Function/1, Trigonometric Function2/1
  Roll_angle(z1)/1 -> Trigonometric Function1/1, Trigonometric Function3/1
  m * g/1 -> Product1/1, Product3/1, Product2/2
  Trigonometric Function2/1 -> Product2/1
  Trigonometric Function3/1 -> Product3/2
  Product3/1 -> Gain/1
  Gain/1 -> Fy_due_to_mass/1
  Product4/1 -> FZ_due_to_mass/1
  Product2/1 -> Fx_due_to_mass/1
  Trigonometric Function1/1 -> Gain1/1
  Gain1/1 -> Product1/2
  Trigonometric Function/1 -> Product4/1
  Product1/1 -> Product4/2

== system PC_Simulator_Lib/Vehicle dynamics/Horizontal_Dyn/Beta_Slip_Angle_calculation ==
  note: this block is to develop the beta
      | slip angle and the absolut speed
      | with which the vehicle travels
      | considering direction of traveling
  Longitudinal_Velocity_Vx : Inport
  Longitudinal_Velocity_Vy : Inport  Port=2
  Bus Creator : BusCreator  Inputs=2
  Divide1 : Product  Inputs=/*
  Divide2 : Product  Inputs=**
  Divide3 : Product  Inputs=**
  Math Function : Math  Operator=sqrt  SaturateOnIntegerOverflow=on
  Sign : Signum
  Sum : Sum
  Trigonometric Function1 : Trigonometry  Operator=atan
  Beta_Slip_Angle : Outport
  absolute_velocity_of_car_with_direction : Outport  Port=2
  wires:
  Longitudinal_Velocity_Vx/1 -> Divide1/1, Divide2/2, Sign/1, Divide2/1
  Divide1/1 -> Trigonometric Function1/1
  Trigonometric Function1/1 -> Beta_Slip_Angle/1
  Longitudinal_Velocity_Vy/1 -> Divide3/1, Divide3/2, Divide1/2
  Divide2/1 -> Sum/1
  Divide3/1 -> Sum/2
  Sum/1 -> Math Function/1
  Sign/1 -> Bus Creator/2
  Bus Creator/1 -> absolute_velocity_of_car_with_direction/1
  Math Function/1 -> Bus Creator/1

== system PC_Simulator_Lib/Vehicle dynamics/Horizontal_Dyn/about_z_axis ==
  note: Yawddot
  Moment _about _Z_axis : Inport
  reset : Inport  Port=2
  1/Inertia_Vertical axis : Gain  Gain=1/Para.VD.Inertia_zz.v  OutDataTypeStr=double
  Integrator1 : Integrator  InitialCondition=Heading_init
  Integrator4 : Integrator  ExternalReset=level
  Yaw_Angular_ACC : Outport
  Yaw_angle_Velcity : Outport  Port=2
  Yaw_angle_(rad) : Outport  Port=3
  wires:
  Moment _about _Z_axis/1 -> 1/Inertia_Vertical axis/1
  1/Inertia_Vertical axis/1 -> Yaw_Angular_ACC/1, Integrator4/1
  Integrator1/1 -> Yaw_angle_(rad)/1
  Integrator4/1 -> Integrator1/1, Yaw_angle_Velcity/1
  reset/1 -> Integrator4/2

== system PC_Simulator_Lib/Vehicle dynamics/Horizontal_Dyn/in_x_direction ==
  note: XDDot
  Force_acting_on_CG_in_x : Inport
  Constant : Constant  Value=eps
  Integrator2 : Integrator  InitialCondition=eps
  Integrator3 : Integrator
  Mass : Gain  Gain=1/Para.VD.Mass.v
  Sum : Sum  Inputs=|++
  Longitudinal_Velocity_Vx : Outport
  Displacement_x : Outport  Port=2
  Acceleration_Ax : Outport  Port=3
  wires:
  Integrator3/1 -> Displacement_x/1
  Mass/1 -> Integrator2/1, Acceleration_Ax/1
  Integrator2/1 -> Integrator3/1, Longitudinal_Velocity_Vx/1
  Force_acting_on_CG_in_x/1 -> Sum/1
  Sum/1 -> Mass/1
  Constant/1 -> Sum/2

== system PC_Simulator_Lib/Vehicle dynamics/Horizontal_Dyn/in_y_direction ==
  note: YDot
  note: Y
  note: YDDot
  Force_acting_on_CG_in_y : Inport
  reset : Inport  Port=2
  Integrator2 : Integrator  ExternalReset=level
  Integrator3 : Integrator
  Mass : Gain  Gain=1/Para.VD.Mass.v
  Lateral_Velocity_Vy : Outport
  Displacement_y : Outport  Port=2
  Acceleration_Ay : Outport  Port=3
  wires:
  Integrator3/1 -> Displacement_y/1
  Force_acting_on_CG_in_y/1 -> Mass/1
  Mass/1 -> Integrator2/1, Acceleration_Ay/1
  Integrator2/1 -> Integrator3/1, Lateral_Velocity_Vy/1
  reset/1 -> Integrator2/2

== system PC_Simulator_Lib/Vehicle dynamics/Horizontal_Dyn/reset ==
  In1 : Inport
  Abs : Abs
  Compare To Constant : simulink/Logic and Bit Operations/Compare To Constant  relop=<=  const=0.5  OutDataTypeStr=boolean
  Out1 : Outport
  wires:
  In1/1 -> Abs/1
  Abs/1 -> Compare To Constant/1
  Compare To Constant/1 -> Out1/1

== system PC_Simulator_Lib/Vehicle dynamics/Horizontal_Dyn/reset1 ==
  In1 : Inport
  Abs : Abs
  Compare To Constant : simulink/Logic and Bit Operations/Compare To Constant  relop=<=  const=0.5  OutDataTypeStr=boolean
  Out1 : Outport
  wires:
  Compare To Constant/1 -> Out1/1
  Abs/1 -> Compare To Constant/1
  In1/1 -> Abs/1

== system PC_Simulator_Lib/Vehicle dynamics/Output_Maping/Subsystem1 ==
  Force_Suspention : Inport
  Bus Creator : BusCreator
  Demux : Demux
  Fz_Wheel[N] : Outport
  wires:
  Force_Suspention/1 -> Demux/1
  Demux/1 -> Bus Creator/1  "Fz_Wheel_FL[N]"
  Demux/2 -> Bus Creator/2  "Fz_Wheel_FR[N]"
  Demux/3 -> Bus Creator/3  "Fz_Wheel_RL[N]"
  Demux/4 -> Bus Creator/4  "Fz_Wheel_RR[N]"
  Bus Creator/1 -> Fz_Wheel[N]/1

== system PC_Simulator_Lib/Vehicle dynamics/Output_Maping/Velocity_Wheels_Maping_Block ==
  Velocity_Wheels_X[m|s] : Inport
  Velocity_Wheels_Y[m|s] : Inport  Port=2
  Bus Creator : BusCreator
  Bus Creator{3..5,7} (4 alike) : BusCreator  Inputs=2
  Demux1 : Demux
  Demux2 : Demux
  Velocity_Wheels[m|s] : Outport
  wires:
  Bus Creator3/1 -> Bus Creator/1  "v_FL[m|s]"
  Bus Creator4/1 -> Bus Creator/2  "v_FR[m|s]"
  Bus Creator5/1 -> Bus Creator/3  "v_RL[m|s]"
  Bus Creator7/1 -> Bus Creator/4  "v_RR[m|s]"
  Demux1/1 -> Bus Creator3/1  "vx_FL[m|s]"
  Demux2/1 -> Bus Creator3/2  "vy_FL[m|s]"
  Demux1/2 -> Bus Creator4/1  "vx_FR[m|s]"
  Demux2/2 -> Bus Creator4/2  "vy_FR[m|s]"
  Demux1/3 -> Bus Creator5/1  "vx_RL[m|s]"
  Demux2/3 -> Bus Creator5/2  "vy_RL[m|s]"
  Demux1/4 -> Bus Creator7/1  "vx_RR[m|s]"
  Demux2/4 -> Bus Creator7/2  "vy_RR"
  Velocity_Wheels_X[m|s]/1 -> Demux1/1
  Velocity_Wheels_Y[m|s]/1 -> Demux2/1
  Bus Creator/1 -> Velocity_Wheels[m|s]/1  "Velocity_Wheels[m|s]"

== system PC_Simulator_Lib/Vehicle dynamics/Vertical_Dyn./Invers_Trangnometric_conv ==
  Vertical_Displacement_Z_vehicle_corners_actual(4) : Inport
  Add3 : Sum  Inputs=++++-
  Constant3 : Constant  Value=-2*Para.VD.Length_Front.v
  Constant4 : Constant  Value=Para.VD.Wheel_Base_Width.v
  Constant5 : Constant  Value=2*Para.VD.Length_Rear.v-2*Para.VD.Length_Front.v
  Demux : Demux
  Divide : Product  Inputs=*/
  Divide1 : Product  Inputs=*/
  Gain1 : Gain  Gain=0.25
  Product3 : Product  RndMeth=Zero
  Subtract3 : Sum  Inputs=+-
  Subtract4 : Sum  Inputs=+-
  Trigonometric Function1 : Trigonometry  Operator=asin
  Trigonometric Function2 : Trigonometry  Operator=asin
  Vertical_Displacement_Z_CG_actual : Outport
  Roll_actual : Outport  Port=2
  Pitch_actual : Outport  Port=3
  wires:
  Vertical_Displacement_Z_vehicle_corners_actual(4)/1 -> Demux/1
  Demux/1 -> Subtract3/1, Subtract4/1, Add3/1
  Demux/3 -> Subtract3/2, Add3/3
  Subtract3/1 -> Divide/1
  Constant3/1 -> Divide/2
  Divide/1 -> Trigonometric Function1/1, Product3/1
  Trigonometric Function1/1 -> Pitch_actual/1
  Demux/2 -> Subtract4/2, Add3/2
  Subtract4/1 -> Divide1/1
  Constant4/1 -> Divide1/2
  Divide1/1 -> Trigonometric Function2/1
  Trigonometric Function2/1 -> Roll_actual/1
  Demux/4 -> Add3/4
  Constant5/1 -> Product3/2
  Product3/1 -> Add3/5
  Add3/1 -> Gain1/1
  Gain1/1 -> Vertical_Displacement_Z_CG_actual/1

== system PC_Simulator_Lib/Vehicle dynamics/Vertical_Dyn./Mass_Distribution ==
  note: Reaction_Force_Front_Wheels
  note: Reaction_Force_Rear_Wheels
  note: FL_Z
  note: FR_Z
  note: RL_Z
  note: RR_Z
  note: Force acting on front wheels = (m*g*Rear_Length)/(Front_Length+Rear_Length)
      | Force acting on Rear wheels = m*g -  (m*g*Rear_Length)/(Front_Length+Rear_Length)
      | the mass are just dividing by the gravity
  Mass*gravity_in_Z : Inport
  Abs : Abs
  Divide : Product  Inputs=*/
  Divide1 : Product  Inputs=*/
  Divide2 : Product  Inputs=*/
  Gain : Gain  Gain=0.5
  Gain1 : Gain  Gain=0.5
  Length_CG_Rear_Wheels : Constant  Value=Para.VD.Length_Rear.v
  Mass*gravity1 : Constant  Value=Para.VD.gravity.v*Para.VD.Mass.v
  Mux : Mux
  Mux1 : Mux
  Product : Product  RndMeth=Zero
  Subtract : Sum  Inputs=+-
  Terminator : Terminator
  Terminator1 : Terminator
  Wheel_Base_Length : Constant  Value=Para.VD.Wheel_Base_Length.v
  gravity : Constant  Value=Para.VD.gravity.v
  Forces_Z_Mass : Outport
  wires:
  Mass*gravity_in_Z/1 -> Abs/1
  Length_CG_Rear_Wheels/1 -> Product/2
  Product/1 -> Divide/1
  Wheel_Base_Length/1 -> Divide/2
  Divide/1 -> Subtract/2, Gain/1
  Subtract/1 -> Gain1/1
  Gain/1 -> Mux/1, Mux/2, Divide1/1
  Gain1/1 -> Mux/3, Mux/4, Divide2/1
  Mux/1 -> Forces_Z_Mass/1
  Divide2/1 -> Mux1/4, Mux1/3
  Divide1/1 -> Mux1/1, Mux1/2
  gravity/1 -> Divide1/2, Divide2/2
  Mass*gravity1/1 -> Terminator1/1
  Mux1/1 -> Terminator/1
  Abs/1 -> Product/1, Subtract/1

== system PC_Simulator_Lib/Vehicle dynamics/Vertical_Dyn./Trangnometric_conv ==
  note: Lf*sin(pitch)
  note: Lr*sin(Pitch)
  note: 0.5*Lt*sin(Roll)
  note: FL
  note: FR
  note: RL
  note: RR
  Vertical_Displacement_Z_CG : Inport
  Pitch : Inport  Port=2
  Roll : Inport  Port=3
  Add : Sum
  Add1 : Sum
  Add2 : Sum
  Constant : Constant  Value=Para.VD.Wheel_Base_Width.v
  Constant1 : Constant  Value=Para.VD.Length_Rear.v
  Constant2 : Constant  Value=Para.VD.Length_Front.v
  Gain : Gain  Gain=0.5
  Mux : Mux
  Product : Product  RndMeth=Zero
  Product1 : Product  RndMeth=Zero
  Product2 : Product  RndMeth=Zero
  Subtract : Sum  Inputs=+-
  Subtract1 : Sum  Inputs=+-
  Subtract2 : Sum  Inputs=+-
  Trigonometric Function : Trigonometry
  Trigonometric Function1 : Trigonometry
  Vertical_Displacement_Z_vehicle_corners(4) : Outport
  wires:
  Mux/1 -> Vertical_Displacement_Z_vehicle_corners(4)/1
  Constant/1 -> Gain/1
  Pitch/1 -> Trigonometric Function/1
  Roll/1 -> Trigonometric Function1/1
  Gain/1 -> Product/2
  Trigonometric Function1/1 -> Product/1
  Trigonometric Function/1 -> Product2/2, Product1/2
  Constant1/1 -> Product2/1
  Constant2/1 -> Product1/1
  Product1/1 -> Subtract/2
  Product2/1 -> Add1/2
  Product/1 -> Add/1, Subtract1/2, Add2/1, Subtract2/2
  Vertical_Displacement_Z_CG/1 -> Subtract/1, Add1/1
  Subtract/1 -> Add/2, Subtract1/1
  Add/1 -> Mux/1
  Subtract1/1 -> Mux/2
  Add1/1 -> Add2/2, Subtract2/1
  Add2/1 -> Mux/3
  Subtract2/1 -> Mux/4

== system PC_Simulator_Lib/Vehicle dynamics/Vertical_Dyn./Vertical_movement ==
  Vertical_Force_CG : Inport
  Moment_Y-axis_CG : Inport  Port=2
  Moment_X-axis_CG : Inport  Port=3
  1/Ixx : Gain  Gain=1/Para.VD.Inertia_xx.v
  1/Iyy : Gain  Gain=1/Para.VD.Inertia_yy.v
  1/mass : Gain  Gain=1/Para.VD.Mass.v
  Integrator{1..6} (6 alike) : Integrator
  Vertical_Displacement_Z_CG : Outport
  Pitch : Outport  Port=2
  Roll : Outport  Port=3
  Vertical_Velocity_Z_CG[m|s] : Outport  Port=4
  wires:
  Vertical_Force_CG/1 -> 1/mass/1
  Moment_Y-axis_CG/1 -> 1/Iyy/1
  Moment_X-axis_CG/1 -> 1/Ixx/1
  1/mass/1 -> Integrator6/1
  Integrator6/1 -> Integrator1/1, Vertical_Velocity_Z_CG[m|s]/1
  Integrator4/1 -> Roll/1
  Integrator2/1 -> Pitch/1
  Integrator3/1 -> Integrator2/1
  Integrator5/1 -> Integrator4/1
  1/Iyy/1 -> Integrator3/1
  1/Ixx/1 -> Integrator5/1
  Integrator1/1 -> Vertical_Displacement_Z_CG/1

== system PC_Simulator_Lib/Vehicle dynamics/Vertical_Dyn./suspention_System ==
  Vertical_Displacement_Z2_vehicle_corners(4) : Inport
  Vertical_Displacement_Z0(4) : Inport  Port=2
  intial_force_from_mass_Wheels(4) : Inport  Port=3
  Demux : Demux
  Demux1 : Demux
  Demux3 : Demux
  Mux{,1..3} (4 alike) : Mux
  Rear_Right_Suspention : Subsystem
  Rear_left_Suspention : Subsystem
  front_left_Suspention : Subsystem
  front_right_Suspention : Subsystem
  Force_Suspention(4) : Outport
  Hight_Suspention(4) : Outport  Port=2
  Z1(4) : Outport  Port=3
  Vertical_Displacement_Z_vehicle_corners_actual(4) : Outport  Port=4
  wires:
  Rear_Right_Suspention/2(Hight_Reer_Right) -> Mux1/4
  Rear_Right_Suspention/1(Force_Suspention_RR) -> Mux/4
  Demux3/4 -> Rear_Right_Suspention/3(intial_force_form_mass_rr)
  Demux1/4 -> Rear_Right_Suspention/2(Vertical_Displacement_Z0)
  Demux/4 -> Rear_Right_Suspention/1(Vertical_Displacement_Z_vehicle_corner_RR)
  Rear_left_Suspention/2(Hight_Reer_left) -> Mux1/3
  intial_force_from_mass_Wheels(4)/1 -> Demux3/1
  Mux1/1 -> Hight_Suspention(4)/1
  Vertical_Displacement_Z0(4)/1 -> Demux1/1
  Vertical_Displacement_Z2_vehicle_corners(4)/1 -> Demux/1
  Mux/1 -> Force_Suspention(4)/1
  Rear_left_Suspention/1(Force_Suspention_RL) -> Mux/3
  Demux/1 -> front_left_Suspention/1(Vertical_Displacement_Z_vehicle_corner_fl)
  Demux/2 -> front_right_Suspention/1(Vertical_Displacement_Z_vehicle_corner_fr)
  Demux/3 -> Rear_left_Suspention/1(Vertical_Displacement_Z_vehicle_corner_Rl)
  Demux1/1 -> front_left_Suspention/2(Vertical_Displacement_Z0)
  Demux1/2 -> front_right_Suspention/2(Vertical_Displacement_Z0)
  Demux1/3 -> Rear_left_Suspention/2(Vertical_Displacement_Z0)
  Demux3/1 -> front_left_Suspention/3(intial_force_form_mass_fl)
  Demux3/2 -> front_right_Suspention/3(intial_force_form_mass_fr)
  Demux3/3 -> Rear_left_Suspention/3(intial_force_form_mass_rl)
  front_left_Suspention/1(Force_Suspention_FL) -> Mux/1
  front_right_Suspention/1(Force_Suspention_FR) -> Mux/2
  front_left_Suspention/2(Hight_front_left) -> Mux1/1, front_right_Suspention/4(Hight_front_left)
  front_right_Suspention/2(Hight_front_right) -> Mux1/2, front_left_Suspention/4(Hight_front_right)
  front_left_Suspention/3(Z1) -> Mux2/1
  front_right_Suspention/3(Z1) -> Mux2/2
  Rear_left_Suspention/3(Z1) -> Mux2/3
  Rear_Right_Suspention/3(Z1) -> Mux2/4
  Mux2/1 -> Z1(4)/1
  Mux3/1 -> Vertical_Displacement_Z_vehicle_corners_actual(4)/1
  front_left_Suspention/4(Z2actual) -> Mux3/1
  front_right_Suspention/4(Z2actual) -> Mux3/2
  Rear_left_Suspention/4(Z2actual) -> Mux3/3
  Rear_Right_Suspention/4(Z2actual) -> Mux3/4

== system PC_Simulator_Lib/Vehicle dynamics/force_from_wheel_cordination_transformation/Steer_model ==
  note: FLxcos+FLysin
  note: FLxsin+FLycos
  note: FRxcos+FRysin
  note: FRxsin+FRycos
  note: To transform the front wheels forces to be calculated in the horizontal block
  note: this block is to find the angle of rotation of
      | the front left and rear wheels
  note: this block is to analyze the
      | forces acting on the wheels
      |  coordination to find thier
      | components on the car coordination
      | -with respect to CAR XY-
  Steering_Angle_HMI_[-1 1] : Inport
  FLx_T : Inport  Port=2
  FRx_T : Inport  Port=3
  FLy_T : Inport  Port=4
  FRy_T : Inport  Port=5
  Force_Analysis : Subsystem
  Steer_Angel_Distribution1 : Subsystem
  FLx : Outport
  FRx : Outport  Port=2
  FLy : Outport  Port=3
  FRy : Outport  Port=4
  FL_Angle : Outport  Port=5
  FR_Angle : Outport  Port=6
  wires:
  Steering_Angle_HMI_[-1 1]/1 -> Steer_Angel_Distribution1/1(Steering_Angle_HMI_[-1 1])
  Force_Analysis/1(FLx) -> FLx/1
  Force_Analysis/2(FLy) -> FLy/1
  Force_Analysis/3(FRx) -> FRx/1
  Force_Analysis/4(FRy) -> FRy/1
  FLx_T/1 -> Force_Analysis/3(FLx_T)
  FRx_T/1 -> Force_Analysis/4(FRx_T)
  FLy_T/1 -> Force_Analysis/5(FLy_T)
  FRy_T/1 -> Force_Analysis/6(FRy_T)
  Steer_Angel_Distribution1/1(FL_Angle) -> FL_Angle/1, Force_Analysis/1(FL_Angle)
  Steer_Angel_Distribution1/2(FR_Angle) -> FR_Angle/1, Force_Analysis/2(FR_Angle)

== system PC_Simulator_Lib/Vehicle dynamics/velocity/R ==
  note: tan(betaCG)
  note: just for test
  slip_angel_at_Rear_left : Inport
  longitudenal_velocity_Vx : Inport  Port=2
  Lateral_velocity_Vy : Inport  Port=3
  Divide2 : Product  Inputs=/*
  Length_CG_Rear_Wheels : Constant  Value=Para.VD.Length_Rear.v
  Product2 : Product  RndMeth=Zero
  Product3 : Product  RndMeth=Zero
  Product4 : Product  RndMeth=Zero
  Rcg : Math  Operator=sqrt  SaturateOnIntegerOverflow=on
  Subtract : Sum  Inputs=+-
  Subtract1 : Sum  Inputs=+-
  Sum3 : Sum  Inputs=|++
  Width_of_Car/2 : Constant  Value=Para.VD.Wheel_Base_Width.v/2
  la : Product  Inputs=*/
  ln : Product  RndMeth=Zero
  tanbetaRL : Trigonometry  Operator=tan
  R_CG : Outport
  wires:
  longitudenal_velocity_Vx/1 -> Divide2/1
  Lateral_velocity_Vy/1 -> Divide2/2
  Divide2/1 -> Subtract1/1, ln/2
  slip_angel_at_Rear_left/1 -> tanbetaRL/1
  Width_of_Car/2/1 -> Product2/1
  tanbetaRL/1 -> Product2/2, Subtract1/2
  Length_CG_Rear_Wheels/1 -> Subtract/1
  Product2/1 -> Subtract/2
  Subtract/1 -> la/1
  Subtract1/1 -> la/2
  la/1 -> ln/1, Product4/1, Product4/2
  ln/1 -> Product3/1, Product3/2
  Product3/1 -> Sum3/1
  Product4/1 -> Sum3/2
  Sum3/1 -> Rcg/1
  Rcg/1 -> R_CG/1
